simulink model "Model_6DOF"  (R2022a)
settings: Solver=FixedStepAuto  StartTime=0.0  StopTime=Tf  FixedStep=0.05  RelTol=1e-3
values from neighbouring files (symbols this model uses):
  Ba_0 = [0 0 0 0 0 0]    [run.m]
  Bv_0 = [-5.14444 0 0 0 0 0]    [run.m]
  Bx_0 = [0 0 -20 0 0 0]    [run.m]
  psi_ref = 0    [run.m]
  Seastate = 0    [run.m]
  Tf = 5000    [run.m]
  v_ref = Bv_0(1)    [run.m]
  z_ref = Bx_0(3)    [run.m]
undefined symbols (not defined in the file or in its folder): Bb, Cp, Cp_prime, dA_BP1, dA_BP2, dA_Hull, dA_PH, dA_Sail, dA_SProot, dA_X1a, dA_X1b, dA_X2a, dA_X2b, dA_X3a, dA_X3b, dA_X4a, dA_X4b, Ixx, Ixy, Ixz, Iyy, Iyz, Izz, Mb, n_BP1, n_BP2, n_Hull, n_PH, n_Sail, n_SProot, n_X2a, n_X2b, n_X3a, n_X4a, n_X4b, nt_BP1, nt_BP2, nt_Hull, nt_PH, nt_Sail, nt_SProot, nt_X1a, nt_X1b, nt_X2a, nt_X2b, nt_X3a, nt_X3b, nt_X4a, nt_X4b, tknots, vt1_BP1, vt1_BP2, vt1_Hull, vt1_PH, vt1_Sail, vt1_SProot, vt1_X1a, vt1_X1b, vt1_X2a, vt1_X2b ... (+39)
libraries: simulink x8
(part 2 of 5)

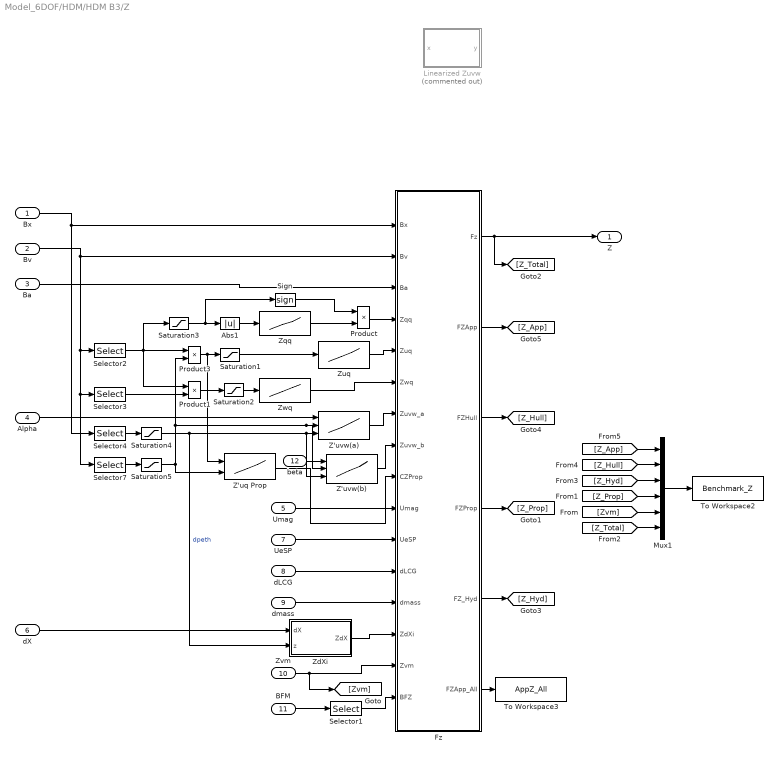
== system Model_6DOF/HDM/HDM B3/Z ==
  Bx : Inport
  Bv : Inport  Port=2
  Ba : Inport  Port=3
  Alpha : Inport  Port=4
  Umag : Inport  Port=5
  dX : Inport  Port=6
  UeSP : Inport  Port=7
  dLCG : Inport  Port=8
  dmass : Inport  Port=9
  Zvm : Inport  Port=10
  BFM : Inport  Port=11
  beta : Inport  Port=12
  Abs1 : Abs  SaturateOnIntegerOverflow=off
  Fz : MATLAB Function  TreatAsAtomicUnit=on
  Linearized Zuvw : MATLAB Function  Commented=on  TreatAsAtomicUnit=on
  Mux1 : Mux  Inputs=6
  Product : Product
  Product1 : Product
  Product3 : Product
  Saturation1 : Saturate  UpperLimit=0.04  LowerLimit=-0.04
  Saturation2 : Saturate  UpperLimit=0.0015  LowerLimit=-0.0015
  Saturation3 : Saturate  UpperLimit=0.02  LowerLimit=-0.02
  Saturation4 : Saturate  UpperLimit=-13.8724  LowerLimit=-35.0624
  Saturation5 : Saturate  UpperLimit=-1.5433E+00  LowerLimit=-5.14444
  Selector1 : Selector  InputPortWidth=6  IndexOptions=Index vector (dialog)  Indices=3  OutputSizes=1
  Selector2 : Selector  InputPortWidth=6  IndexOptions=Index vector (dialog)  Indices=5  OutputSizes=1
  Selector3 : Selector  InputPortWidth=6  IndexOptions=Index vector (dialog)  Indices=3  OutputSizes=1
  Selector4 : Selector  InputPortWidth=6  IndexOptions=Index vector (dialog)  Indices=3  OutputSizes=1
  Selector7 : Selector  InputPortWidth=6  IndexOptions=Index vector (dialog)  Indices=1  OutputSizes=1
  Sign : Signum
  To Workspace2 : ToWorkspace  VariableName=Benchmark_Z  SaveFormat=Timeseries  SampleTime=-1
  To Workspace3 : ToWorkspace  VariableName=AppZ_All  SaveFormat=Timeseries  SampleTime=-1
  Z'uq Prop : Lookup_n-D  BreakpointsForDimension1=|  BreakpointsForDimension2=[-7.71666 -5.14444 -3.086664 -1.543332]  Table=|  InternalRulePriority=Speed  RndMeth=Simplest
      BreakpointsForDimension1=|
      | [-2.0E-01
      | -1.5E-01
      | -1.0E-01
      | -5.0E-02
      | 0.0E+00
      | 5.0E-02
      | 1.0E-01
      | 1.5E-01
      | 2.0E-01
      | ]
      Table=|
      | reshape([1.3913E-04
      | 1.0452E-04
      | 6.9900E-05
      | 3.5283E-05
      | 6.6700E-07
      | -3.3949E-05
      | -6.8566E-05
      | -1.0318E-04
      | -1.3780E-04
      | 2.8914E-04
      | 2.1702E-04
      | 1.4490E-04
      | 7.2785E-05
      | 6.6700E-07
      | -7.1451E-05
      | -1.4357E-04
      | -2.1569E-04
      | -2.8780E-04
      | 1.1606E-04
      | 8.7208E-05
      | 5.8361E-05
      | 2.9514E-05
      | 6.6700E-07
      | -2.8180E-05
      | -5.7027E-05
      | -8.5874E-05
      | -1.1472E-04
      | 1.1606E-04
      | 8.7208E-05
      | 5.8361E-05
      | 2.9514E-05
      | 6.6700E-07
      | -2.8180E-05
      | -5.7027E-05
      | -8.5874E-05
      | -1.1472E-04],[9,4])
      settings: InputPortMap=u0,u1
  Z'uvw(a) : Lookup_n-D  NumberOfTableDimensions=3  BreakpointsForDimension1=|  BreakpointsForDimension2=|  BreakpointsForDimension3=|  Table=|  InternalRulePriority=Speed  RndMeth=Simplest
      BreakpointsForDimension1=|
      | [-12
      | -8
      | -4
      | 0
      | 4
      | 8
      | 12]
      BreakpointsForDimension2=|
      | [-5.1444E+00
      | -3.0866E+00
      | -1.5433E+00
      | ]
      Table=|
      | reshape([-3.82587E-03
      | -2.42543E-03
      | -1.05453E-03
      | 1.94202E-04
      | 1.48991E-03
      | 3.04047E-03
      | 4.14104E-03
      | -3.76348E-03
      | -2.38508E-03
      | -9.82619E-04
      | 1.94202E-04
      | 1.47560E-03
      | 3.02863E-03
      | 4.06663E-03
      | -3.75964E-03
      | -2.29001E-03
      | -8.34074E-04
      | 1.94202E-04
      | 1.38956E-03
      | 2.91153E-03
      | 4.15251E-03
      | -3.11218E-03
      | -1.80502E-03
      | -4.97855E-04
      | 8.09305E-04
      | 2.11647E-03
      | 3.42363E-03
      | 4.73079E-03
      | -2.62573E-03
      | -1.48072E-03
      | -3.35708E-04
      | 8.09305E-04
      | 1.95432E-03
      | 3.09933E-03
      | 4.24434E-03
      | -2.06413E-03
      | -1.10632E-03
      | -1.48507E-04
      | 8.09305E-04
      | 1.76712E-03
      | 2.72493E-03
      | 3.68274E-03
      | -3.09997E-03
      | -1.76300E-03
      | -4.26025E-04
      | 9.10947E-04
      | 2.24792E-03
      | 3.58489E-03
      | 4.92186E-03
      | -2.49055E-03
      | -1.35672E-03
      | -2.22886E-04
      | 9.10947E-04
      | 2.04478E-03
      | 3.17861E-03
      | 4.31245E-03
      | -2.64104E-03
      | -1.45704E-03
      | -2.73048E-04
      | 9.10947E-04
      | 2.09494E-03
      | 3.27894E-03
      | 4.46293E-03
      | -0.003059752
      | -0.001711935
      | -0.000364117
      | 0.0009837
      | 0.002331518
      | 0.003679335
      | 0.005027153
      | -0.002351082
      | -0.0012256
      | -0.000100118
      | 0.0009837
      | 0.002109182
      | 0.003234664
      | 0.004360146
      | -0.001725739
      | -0.000822593
      | 8.05539E-05
      | 0.0009837
      | 0.001886847
      | 0.002789993
      | 0.00369314],[7,3,4])
      BreakpointsForDimension3=|
      | [-35.0624 -18.3724 -15.3724 -13.8724
      | ]
      settings: InputPortMap=u0,u1,u2
  Z'uvw(b) : Lookup_n-D  NumberOfTableDimensions=3  BreakpointsForDimension1=|  BreakpointsForDimension2=|  BreakpointsForDimension3=|  Table=|  InternalRulePriority=Speed  RndMeth=Simplest
      BreakpointsForDimension1=|
      | [0
      | 4
      | 8
      | 12]
      BreakpointsForDimension2=|
      | [-5.1444E+00
      | -3.0866E+00
      | -1.5433E+00
      | ]
      Table=|
      | reshape([0.0000000E+00
      | -5.9986916E-04
      | -2.7503348E-03
      | -5.0777589E-03
      | 0.0000000E+00
      | -6.0654884E-04
      | -2.4512564E-03
      | -5.2464901E-03
      | 0.0000000E+00
      | -7.6137528E-04
      | -2.4084463E-03
      | -5.2118678E-03
      | 0.0000000E+00
      | -8.2427914E-04
      | -2.5250249E-03
      | -5.3103563E-03
      | 0.0000000E+00
      | -8.1036019E-04
      | -2.5315266E-03
      | -5.5141459E-03
      | 0.0000000E+00
      | -7.9799041E-04
      | -2.5595242E-03
      | -5.2319004E-03
      | 0.0000000E+00
      | -8.6989011E-04
      | -2.5865820E-03
      | -5.6151595E-03
      | 0.0000000E+00
      | -8.4361582E-04
      | -2.6124115E-03
      | -5.7143353E-03
      | 0.0000000E+00
      | -8.2567611E-04
      | -2.6088331E-03
      | -5.6150660E-03
      | 0.0000000E+00
      | -9.1003224E-04
      | -2.7683191E-03
      | -6.0189061E-03
      | 0.0000000E+00
      | -8.4211433E-04
      | -2.5899187E-03
      | -5.7497784E-03
      | 0.0000000E+00
      | -8.2014014E-04
      | -2.4092466E-03
      | -5.6643347E-03],[4,3,4])
      BreakpointsForDimension3=|
      | [-35.0624 -18.3724 -15.3724 -13.8724
      | ]
      settings: InputPortMap=u0,u1,u2
  ZdXi : Subsystem
  Zqq : Lookup_n-D  NumberOfTableDimensions=1  BreakpointsForDimension1=|  Table=|  InternalRulePriority=Speed  RndMeth=Simplest
      BreakpointsForDimension1=|
      | [0.000127901
      | 0.000383704
      | 0.000639507
      | 0.001279013
      | 0.002558026
      | ]
      Table=|
      | [-1.5611E-03
      | -1.0379E-04
      | 3.9238E-05
      | 1.1475E-04
      | 1.3579E-04
      | ]
  Zuq : Lookup_n-D  NumberOfTableDimensions=1  BreakpointsForDimension1=|  Table=|  InternalRulePriority=Speed  RndMeth=Simplest
      BreakpointsForDimension1=|
      | [-0.04
      | -0.03
      | -0.02
      | -0.01
      | -0.005
      | -0.002
      | 0.002
      | 0.005
      | 0.01
      | 0.02
      | 0.03
      | 0.04
      | ]
      Table=|
      | [-9.8908E-03
      | -9.0784E-03
      | -8.9566E-03
      | -1.0733E-02
      | -1.4141E-02
      | -2.4189E-02
      | -6.5605E-03
      | -7.1594E-03
      | -7.6366E-03
      | -7.9008E-03
      | -6.1794E-03
      | -6.1029E-03
      | ]
  Zwq : Lookup_n-D  NumberOfTableDimensions=1  BreakpointsForDimension1=|  Table=|  InternalRulePriority=Speed  RndMeth=Simplest
      BreakpointsForDimension1=|
      | [-0.0015
      | -0.0012
      | -0.0009
      | -0.0006
      | -0.0003
      | -0.0001
      | 0.0001
      | 0.0003
      | 0.0006
      | 0.0009
      | 0.0012
      | 0.0015]
      Table=|
      | [-2.9784E-01
      | -2.6725E-01
      | -2.3292E-01
      | -2.0077E-01
      | -1.1489E-01
      | -7.6673E-03
      | -7.5516E-03
      | -1.1617E-01
      | -2.0077E-01
      | -2.9128E-01
      | -3.5974E-01
      | -4.7839E-01]
  Z : Outport
  wires:
  Selector4/1 -> Saturation4/1
  Zvm/1 -> Fz/15(Zvm), [Zvm]
  Ba/1 -> Fz/3(Ba)
  Zuq/1 -> Fz/5(Zuq)
  Fz/1(Fz) -> Z/1, [Z_Total]
  Saturation3/1 -> Abs1/1, Sign/1
  Saturation2/1 -> Zwq/1
  Saturation1/1 -> Zuq/1
  dX/1 -> ZdXi/1(dX)
  dmass/1 -> Fz/13(dmass)
  dLCG/1 -> Fz/12(dLCG)
  Product1/1 -> Saturation2/1
  Selector3/1 -> Product1/2
  UeSP/1 -> Fz/11(UeSP)
  Product3/1 -> Saturation1/1, Z'uq Prop/1
  Bx/1 -> Fz/1(Bx), Selector4/1
  Umag/1 -> Fz/10(Umag)
  Bv/1 -> Fz/2(Bv), Selector2/1, Selector3/1, Selector7/1
  Alpha/1 -> Z'uvw(a)/1
  Selector2/1 -> Product3/1, Product1/1, Saturation3/1
  Zwq/1 -> Fz/6(Zwq)
  Z'uq Prop/1 -> Fz/9(CZProp)
  Zqq/1 -> Product/2
  Z'uvw(a)/1 -> Fz/7(Zuvw_a)
  BFM/1 -> Selector1/1
  Selector1/1 -> Fz/16(BFZ)
  ZdXi/1(ZdX) -> Fz/14(ZdXi)
  [Z_Hull] -> Mux1/2
  [Z_App] -> Mux1/1
  Mux1/1 -> To Workspace2/1
  [Z_Prop] -> Mux1/4
  [Z_Total] -> Mux1/6
  [Z_Hyd] -> Mux1/3
  [Zvm] -> Mux1/5
  Fz/2(FZApp) -> [Z_App]
  Fz/3(FZHull) -> [Z_Hull]
  Fz/4(FZProp) -> [Z_Prop]
  Fz/5(FZ_Hyd) -> [Z_Hyd]
  Saturation4/1 -> Z'uvw(b)/3, Z'uvw(a)/3, ZdXi/2(z)  "dpeth"
  Saturation5/1 -> Product3/2, Z'uvw(a)/2, Z'uvw(b)/2, Z'uq Prop/2
  Selector7/1 -> Saturation5/1
  Fz/6(FZApp_All) -> To Workspace3/1
  Abs1/1 -> Zqq/1
  Sign/1 -> Product/1
  Product/1 -> Fz/4(Zqq)
  Z'uvw(b)/1 -> Fz/8(Zuvw_b)
  beta/1 -> Z'uvw(b)/1

== system Model_6DOF/HDM/Integration and Coord. Transfrom/Coordinate Transform ==
  Bv : Inport
  Integrator : Integrator  InitialCondition=Bx_0
  MATLAB Function2 : MATLAB Function  TreatAsAtomicUnit=on
  X_earth : Outport  VectorParamsAs1DForOutWhenUnconnected=off
  wires:
  Bv/1 -> MATLAB Function2/2(Bv)
  MATLAB Function2/1(out) -> Integrator/1
  Integrator/1 -> X_earth/1, MATLAB Function2/1(Bx)

== system Model_6DOF/HDM/Integration and Coord. Transfrom/Rigid Body Motion ==
  F_hyd : Inport
  Bx : Inport  Port=2
  Demux : Demux  Outputs=6
  Demux1 : Demux  Outputs=6
  Demux2 : Demux  Outputs=5
  Gain2 : Gain
  Integrator : Integrator  InitialCondition=Bv_0
  MATLAB Function2 : MATLAB Function  TreatAsAtomicUnit=on
  Memory1 : Memory  InitialCondition=Ba_0
  Mux1 : Mux  Inputs=6
  Mux2 : Mux  Inputs=5
  Bv : Outport  VectorParamsAs1DForOutWhenUnconnected=off
  Ba : Outport  Port=2  VectorParamsAs1DForOutWhenUnconnected=off
  wires:
  Bx/1 -> MATLAB Function2/7(bx)
  MATLAB Function2/1(out) -> Integrator/1, Memory1/1
  Integrator/1 -> MATLAB Function2/8(bv), Demux1/1
  Memory1/1 -> Ba/1
  Demux/1 -> MATLAB Function2/1(X)
  Demux/2 -> MATLAB Function2/2(Y)
  Demux/3 -> MATLAB Function2/3(Z)
  Demux/4 -> MATLAB Function2/4(K)
  Demux/5 -> MATLAB Function2/5(M)
  Demux/6 -> MATLAB Function2/6(N)
  F_hyd/1 -> Demux/1
  Demux2/3 -> Mux1/4
  Demux1/3 -> Mux2/2
  Mux2/1 -> Gain2/1
  Demux2/5 -> Mux1/6
  Demux2/2 -> Mux1/3
  Demux2/4 -> Mux1/5
  Demux1/1 -> Mux1/1
  Demux2/1 -> Mux1/2
  Demux1/5 -> Mux2/4
  Demux1/6 -> Mux2/5
  Demux1/4 -> Mux2/3
  Demux1/2 -> Mux2/1
  Gain2/1 -> Demux2/1
  Mux1/1 -> Bv/1

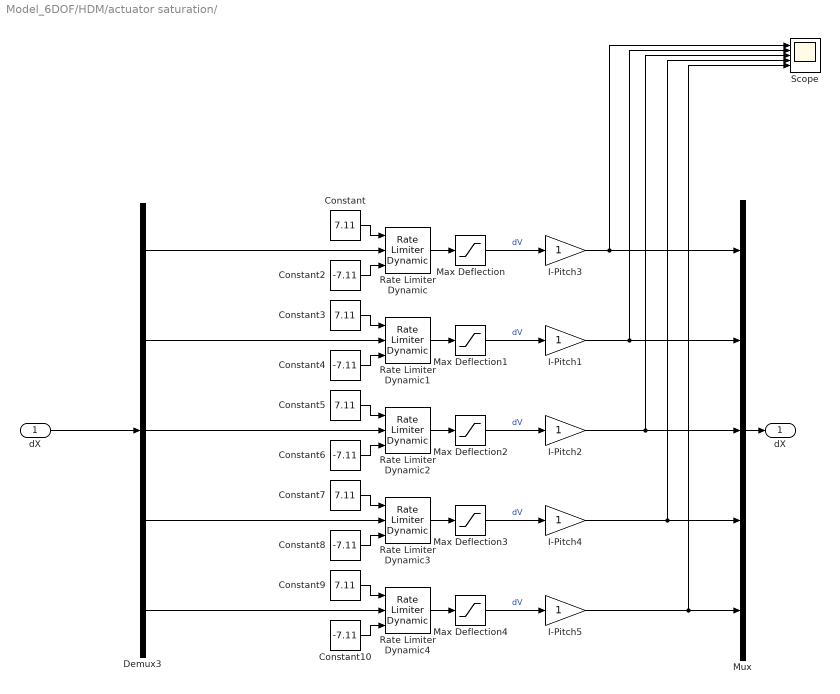
== system Model_6DOF/HDM/actuator saturation/  ==
  "dX " : Inport
  Constant{,3,5,7,9} (5 alike) : Constant  Value=7.11
  Constant{2,4,6,8,10} (5 alike) : Constant  Value=-7.11
  Demux3 : Demux  Outputs=5
  I-Pitch{1..5} (5 alike) : Gain
  Max Deflection{,1..4} (5 alike) : Saturate  UpperLimit=30  LowerLimit=-30
  Mux : Mux  Inputs=5
  Rate Limiter Dynamic{,1..4} (5 alike) : simulink/Discontinuities/Rate Limiter Dynamic
  Scope : Scope  NumInputPorts=5
  dX : Outport
  wires:
  I-Pitch2/1 -> Scope/3, Mux/3
  Constant2/1 -> Rate Limiter Dynamic/3
  Constant9/1 -> Rate Limiter Dynamic4/1
  Demux3/1 -> Rate Limiter Dynamic/2
  Max Deflection/1 -> I-Pitch3/1  "dV"
  Demux3/3 -> Rate Limiter Dynamic2/2
  Demux3/5 -> Rate Limiter Dynamic4/2
  Constant3/1 -> Rate Limiter Dynamic1/1
  Demux3/4 -> Rate Limiter Dynamic3/2
  Demux3/2 -> Rate Limiter Dynamic1/2
  Constant10/1 -> Rate Limiter Dynamic4/3
  Rate Limiter Dynamic/1 -> Max Deflection/1
  I-Pitch5/1 -> Scope/5, Mux/5
  Rate Limiter Dynamic4/1 -> Max Deflection4/1
  Max Deflection2/1 -> I-Pitch2/1  "dV"
  I-Pitch1/1 -> Scope/2, Mux/2
  Constant4/1 -> Rate Limiter Dynamic1/3
  I-Pitch3/1 -> Scope/1, Mux/1
  I-Pitch4/1 -> Scope/4, Mux/4
  Constant6/1 -> Rate Limiter Dynamic2/3
  Rate Limiter Dynamic1/1 -> Max Deflection1/1
  Constant/1 -> Rate Limiter Dynamic/1
  Rate Limiter Dynamic2/1 -> Max Deflection2/1
  Max Deflection1/1 -> I-Pitch1/1  "dV"
  Constant5/1 -> Rate Limiter Dynamic2/1
  Max Deflection3/1 -> I-Pitch4/1  "dV"
  "dX "/1 -> Demux3/1
  Constant8/1 -> Rate Limiter Dynamic3/3
  Max Deflection4/1 -> I-Pitch5/1  "dV"
  Constant7/1 -> Rate Limiter Dynamic3/1
  Mux/1 -> dX/1
  Rate Limiter Dynamic3/1 -> Max Deflection3/1

== system Model_6DOF/HDM/actuator saturation/    ==
  "n " : Inport
  Rate Limiter Dynamic : simulink/Discontinuities/Rate Limiter Dynamic
  Rate Max : Constant  Value=14.65
  Rate Min : Constant  Value=-14.65
  Saturation6 : Saturate  UpperLimit=10  LowerLimit=0.01
  n : Outport
  wires:
  "n "/1 -> Rate Limiter Dynamic/2
  Rate Min/1 -> Rate Limiter Dynamic/3
  Rate Limiter Dynamic/1 -> Saturation6/1
  Rate Max/1 -> Rate Limiter Dynamic/1
  Saturation6/1 -> n/1

== system Model_6DOF/HDM/actuator saturation/Subsystem1 ==
  dLCG : Inport
  " LCG Change Saturation" : Saturate
  Lower Rate limit : Constant  Value=-5.83e-4
  Rate Limiter Dynamic : simulink/Discontinuities/Rate Limiter Dynamic
  Upper Rate limit : Constant  Value=5.83e-4
  dLCG (m) : Outport
  wires:
  " LCG Change Saturation"/1 -> dLCG (m)/1  "dLCG (m)"
  Rate Limiter Dynamic/1 -> " LCG Change Saturation"/1  "dLCG (m)"
  Lower Rate limit/1 -> Rate Limiter Dynamic/3
  Upper Rate limit/1 -> Rate Limiter Dynamic/1
  dLCG/1 -> Rate Limiter Dynamic/2

== system Model_6DOF/HDM/actuator saturation/Subsystem2 ==
  dmass : Inport
  Constant2 : Constant  Value=100
  Constant3 : Constant  Value=-100
  Max Mass Change : Saturate  UpperLimit=20000  LowerLimit=-20000
  Rate Limiter Dynamic1 : simulink/Discontinuities/Rate Limiter Dynamic
  dmass (kg) : Outport
  wires:
  Constant3/1 -> Rate Limiter Dynamic1/3
  Rate Limiter Dynamic1/1 -> Max Mass Change/1  "dmass (kg)"
  Constant2/1 -> Rate Limiter Dynamic1/1
  dmass/1 -> Rate Limiter Dynamic1/2
  Max Mass Change/1 -> dmass (kg)/1  "dmass (kg)"

== system Model_6DOF/HDM/HDM B3/K/KdXi ==
  dX : Inport
  UeX : Inport  Port=2
  z : Inport  Port=3
  KdX1 : Lookup_n-D  NumberOfTableDimensions=3  BreakpointsForDimension1=[-10 0 10]  BreakpointsForDimension2=|  BreakpointsForDimension3=[-5.14444 -3.08666664 -1.54332]  Table=|  InternalRulePriority=Speed  RndMeth=Simplest
      BreakpointsForDimension2=|
      | [-36.4062987
      | -18.4062987
      | -15.4062987
      | -13.9062987]
      Table=|
      | reshape([-3.9047E-05
      | 4.5684E-07
      | 3.9769E-05
      | -3.8309E-05
      | 1.2643E-06
      | 4.0809E-05
      | -3.0256E-05
      | 1.2643E-06
      | 4.8387E-05
      | -3.7558E-05
      | 2.1545E-06
      | 4.2083E-05
      | -3.9057E-05
      | 3.6064E-07
      | 3.9562E-05
      | -3.8473E-05
      | 1.0476E-06
      | 4.0437E-05
      | -3.0256E-05
      | 1.4418E-06
      | 4.8387E-05
      | -3.7906E-05
      | 1.7415E-06
      | 4.1434E-05
      | -3.8945E-05
      | 2.8249E-07
      | 3.9429E-05
      | -3.8396E-05
      | 9.1134E-07
      | 4.0237E-05
      | -3.8190E-05
      | 9.1134E-07
      | 4.0733E-05
      | -3.7932E-05
      | 1.5343E-06
      | 4.1020E-05
      | ],[3,4,3])
      settings: InputPortMap=u0,u1,u2
  KdX2 : Lookup_n-D  NumberOfTableDimensions=3  BreakpointsForDimension1=[-10 0 10]  BreakpointsForDimension2=|  BreakpointsForDimension3=[-5.14444 -3.08666664 -1.54332]  Table=|  InternalRulePriority=Speed  RndMeth=Simplest
      BreakpointsForDimension2=|
      | [-36.4062987
      | -18.4062987
      | -15.4062987
      | -13.9062987]
      Table=|
      | reshape([-3.5775E-05
      | -2.4080E-07
      | 3.3150E-05
      | -3.4263E-05
      | 1.2268E-06
      | 3.5342E-05
      | -2.3577E-05
      | 1.2268E-06
      | 4.6338E-05
      | -3.2368E-05
      | 3.5682E-06
      | 3.9469E-05
      | -3.5785E-05
      | -3.3131E-07
      | 3.3067E-05
      | -3.4544E-05
      | 8.9010E-07
      | 3.4889E-05
      | -2.3577E-05
      | 1.7076E-06
      | 4.6338E-05
      | -3.3141E-05
      | 2.4187E-06
      | 3.7389E-05
      | -3.5809E-05
      | -5.7189E-07
      | 3.3046E-05
      | -3.4706E-05
      | 4.2723E-07
      | 3.4588E-05
      | -3.4017E-05
      | 4.2723E-07
      | 3.5657E-05
      | -3.3562E-05
      | 1.6134E-06
      | 3.6605E-05
      | ],[3,4,3])
      settings: InputPortMap=u0,u1,u2
  KdX3 : Lookup_n-D  NumberOfTableDimensions=3  BreakpointsForDimension1=[-10 0 10]  BreakpointsForDimension2=|  BreakpointsForDimension3=[-5.14444 -3.08666664 -1.54332]  Table=|  InternalRulePriority=Speed  RndMeth=Simplest
      BreakpointsForDimension2=|
      | [-36.4062987
      | -18.4062987
      | -15.4062987
      | -13.9062987]
      Table=|
      | reshape([-4.3139E-05
      | 1.7292E-07
      | 4.5001E-05
      | -4.4081E-05
      | -1.2796E-06
      | 4.2448E-05
      | -4.9749E-05
      | -1.2796E-06
      | 2.6691E-05
      | -4.5613E-05
      | -3.5861E-06
      | 3.8362E-05
      | -4.2707E-05
      | 2.7384E-07
      | 4.4575E-05
      | -4.3360E-05
      | -9.3523E-07
      | 4.2465E-05
      | -4.9749E-05
      | -1.7362E-06
      | 2.6691E-05
      | -4.4279E-05
      | -2.4363E-06
      | 3.9821E-05
      | -4.1687E-05
      | 5.3371E-07
      | 4.3082E-05
      | -4.2289E-05
      | -4.5361E-07
      | 4.1207E-05
      | -4.2616E-05
      | -4.5361E-07
      | 4.0204E-05
      | -4.2521E-05
      | -1.6159E-06
      | 3.9463E-05
      | ],[3,4,3])
      settings: InputPortMap=u0,u1,u2
  KdX4 : Lookup_n-D  NumberOfTableDimensions=3  BreakpointsForDimension1=[-10 0 10]  BreakpointsForDimension2=|  BreakpointsForDimension3=[-5.14444 -3.08666664 -1.54332]  Table=|  InternalRulePriority=Speed  RndMeth=Simplest
      BreakpointsForDimension2=|
      | [-36.4062987
      | -18.4062987
      | -15.4062987
      | -13.9062987]
      Table=|
      | reshape([-4.0969E-05
      | -4.5313E-07
      | 4.0019E-05
      | -4.1787E-05
      | -1.2714E-06
      | 3.9006E-05
      | -4.8908E-05
      | -1.2714E-06
      | 3.0663E-05
      | -4.2681E-05
      | -2.1920E-06
      | 3.7920E-05
      | -4.0777E-05
      | -3.6185E-07
      | 4.0047E-05
      | -4.1470E-05
      | -1.0577E-06
      | 3.9147E-05
      | -4.8908E-05
      | -1.4679E-06
      | 3.0663E-05
      | -4.2187E-05
      | -1.7779E-06
      | 3.8312E-05
      | -4.0496E-05
      | -2.8854E-07
      | 4.0049E-05
      | -4.1082E-05
      | -9.2714E-07
      | 3.9223E-05
      | -4.1472E-05
      | -9.2714E-07
      | 3.8784E-05
      | -4.1733E-05
      | -1.5768E-06
      | 3.8383E-05
      | ],[3,4,3])
      settings: InputPortMap=u0,u1,u2
  Mux : Mux
  Selector1 : Selector  InputPortWidth=5  IndexOptions=Index vector (dialog)  Indices=2  OutputSizes=1
  Selector2 : Selector  InputPortWidth=5  IndexOptions=Index vector (dialog)  Indices=3  OutputSizes=1
  Selector3 : Selector  InputPortWidth=5  IndexOptions=Index vector (dialog)  Indices=4  OutputSizes=1
  Selector4 : Selector  InputPortWidth=5  IndexOptions=Index vector (dialog)  Indices=1  OutputSizes=1
  Selector5 : Selector  InputPortWidth=5  IndexOptions=Index vector (dialog)  Indices=2  OutputSizes=1
  Selector6 : Selector  InputPortWidth=5  IndexOptions=Index vector (dialog)  Indices=3  OutputSizes=1
  Selector7 : Selector  InputPortWidth=5  IndexOptions=Index vector (dialog)  Indices=1  OutputSizes=1
  Selector8 : Selector  InputPortWidth=5  IndexOptions=Index vector (dialog)  Indices=4  OutputSizes=1
  KdXi : Outport
  wires:
  dX/1 -> Selector1/1, Selector3/1, Selector2/1, Selector7/1
  Selector7/1 -> KdX1/1
  Mux/1 -> KdXi/1
  z/1 -> KdX4/2, KdX3/2, KdX2/2, KdX1/2
  KdX1/1 -> Mux/1
  KdX2/1 -> Mux/2
  KdX3/1 -> Mux/3
  KdX4/1 -> Mux/4
  Selector1/1 -> KdX2/1
  Selector2/1 -> KdX3/1
  Selector3/1 -> KdX4/1
  UeX/1 -> Selector6/1, Selector8/1, Selector5/1, Selector4/1
  Selector4/1 -> KdX1/3
  Selector8/1 -> KdX4/3
  Selector6/1 -> KdX3/3
  Selector5/1 -> KdX2/3

== system Model_6DOF/HDM/HDM B3/M/Mdxi ==
  dX : Inport
  z : Inport  Port=2
  Demux6 : Demux  Outputs=5
  Gain{,1..4} (5 alike) : Gain
  Mux : Mux  Inputs=5
  ZudX1 q+1 : Lookup_n-D  BreakpointsForDimension1=[-30 -20 -10 0 10 20 30]  BreakpointsForDimension2=[-35.0624 -15.3724 -13.8724]  BreakpointsForDimension3=[-5.14444 -3.08666664 -1.54332]  Table=|  InternalRulePriority=Speed  RndMeth=Simplest
      | reshape([0.000594819
      | 0.000394915
      | 0.000195011
      | -4.89222E-06
      | -0.000204796
      | -0.0004047
      | -0.000604603
      | 0.000596203
      | 0.000392018
      | 0.000187833
      | -1.6352E-05
      | -0.000220537
      | -0.000424722
      | -0.000628907
      | 0.000582351
      | 0.000381446
      | 0.000180542
      | -2.03625E-05
      | -0.000221267
      | -0.000422171
      | -0.000623076
      | ],[7,3])
      settings: InputPortMap=u0,u1
  ZudX1 q+2 : Lookup_n-D  BreakpointsForDimension1=[-30 -20 -10 0 10 20 30]  BreakpointsForDimension2=[-35.0624 -15.3724 -13.8724]  BreakpointsForDimension3=[-5.14444 -3.08666664 -1.54332]  Table=|  InternalRulePriority=Speed  RndMeth=Simplest
      | reshape([0.000583784
      | 0.000394316
      | 0.000204847
      | 1.53782E-05
      | -0.000174091
      | -0.000363559
      | -0.000553028
      | 0.00056228
      | 0.000374724
      | 0.000187169
      | -3.86644E-07
      | -0.000187942
      | -0.000375498
      | -0.000563053
      | 0.000546298
      | 0.000362052
      | 0.000177806
      | -6.43933E-06
      | -0.000190685
      | -0.000374931
      | -0.000559176],[7,3])
      settings: InputPortMap=u0,u1
  ZudX1 q+3 : Lookup_n-D  BreakpointsForDimension1=[-30 -20 -10 0 10 20 30]  BreakpointsForDimension2=[-35.0624 -15.3724 -13.8724]  BreakpointsForDimension3=[-5.14444 -3.08666664 -1.54332]  Table=|  InternalRulePriority=Speed  RndMeth=Simplest
      | reshape([-0.000586989
      | -0.000395541
      | -0.000204094
      | -1.26467E-05
      | 0.000178801
      | 0.000370248
      | 0.000561695
      | -0.000568868
      | -0.000379268
      | -0.000189669
      | -6.86388E-08
      | 0.000189531
      | 0.000379131
      | 0.000568731
      | -0.000565299
      | -0.000378949
      | -0.000192598
      | -6.24776E-06
      | 0.000180103
      | 0.000366453
      | 0.000552804],[7,3])
      settings: InputPortMap=u0,u1
  ZudX1 q+4 : Lookup_n-D  BreakpointsForDimension1=[-30 -20 -10 0 10 20 30]  BreakpointsForDimension2=[-35.0624 -15.3724 -13.8724]  BreakpointsForDimension3=[-5.14444 -3.08666664 -1.54332]  Table=|  InternalRulePriority=Speed  RndMeth=Simplest
      | reshape([-0.000638396
      | -0.000426715
      | -0.000215035
      | -3.35454E-06
      | 0.000208326
      | 0.000420006
      | 0.000631687
      | -0.000598951
      | -0.000393944
      | -0.000188937
      | 1.60698E-05
      | 0.000221077
      | 0.000426084
      | 0.000631091
      | -0.000622514
      | -0.000421726
      | -0.000220939
      | -2.01522E-05
      | 0.000180635
      | 0.000381422
      | 0.000582209],[7,3])
      settings: InputPortMap=u0,u1
  ZudX1 q+5 : Lookup_n-D  BreakpointsForDimension1=[-30 -20 -10 0 10 20 30]  BreakpointsForDimension2=[-35.0624 -15.3724 -13.8724]  BreakpointsForDimension3=[-35.0624 -15.3724 -13.8724]  Table=|  InternalRulePriority=Speed  RndMeth=Simplest
      | reshape([-0.000461714
      | -0.000296336
      | -0.000130959
      | 3.44194E-05
      | 0.000199797
      | 0.000365175
      | 0.000530553
      | -0.000503641
      | -0.000327652
      | -0.000151663
      | 2.43257E-05
      | 0.000200315
      | 0.000376303
      | 0.000552292
      | -0.000536558
      | -0.000356664
      | -0.00017677
      | 3.1235E-06
      | 0.000183017
      | 0.000362911
      | 0.000542805],[7,3])
      settings: InputPortMap=u0,u1
  MdX : Outport
  wires:
  Demux6/5 -> ZudX1 q+5/1
  Demux6/4 -> ZudX1 q+4/1
  Demux6/3 -> ZudX1 q+3/1
  Demux6/2 -> ZudX1 q+2/1
  ZudX1 q+4/1 -> Gain1/1
  ZudX1 q+3/1 -> Gain2/1
  ZudX1 q+2/1 -> Gain3/1
  ZudX1 q+1/1 -> Gain/1
  ZudX1 q+5/1 -> Gain4/1
  z/1 -> ZudX1 q+5/2, ZudX1 q+4/2, ZudX1 q+3/2, ZudX1 q+2/2, ZudX1 q+1/2
  Mux/1 -> MdX/1
  Demux6/1 -> ZudX1 q+1/1
  dX/1 -> Demux6/1
  Gain/1 -> Mux/1
  Gain3/1 -> Mux/2
  Gain2/1 -> Mux/3
  Gain1/1 -> Mux/4
  Gain4/1 -> Mux/5

== system Model_6DOF/HDM/HDM B3/N/NdXi ==
  dX : Inport
  z : Inport  Port=2
  Mux : Mux
  NdX1 : Lookup_n-D  BreakpointsForDimension1=[-10 0 10]  BreakpointsForDimension2=|  BreakpointsForDimension3=[-5.14444 -3.08666664 -1.54332]  Table=|  InternalRulePriority=Speed  RndMeth=Simplest
      BreakpointsForDimension2=|
      | [-36.4062987
      | -18.4062987
      | -15.4062987
      | -13.9062987]
      Table=|
      | reshape([-8.13475E-05
      | -3.25752E-06
      | 6.9363E-05
      | -8.00129E-05
      | -1.7093E-06
      | 7.14001E-05
      | -6.46417E-05
      | -1.7093E-06
      | 8.57128E-05
      | -7.85432E-05
      | -1.19372E-08
      | 7.37459E-05],[3,4])
      settings: InputPortMap=u0,u1
  NdX2 : Lookup_n-D  BreakpointsForDimension1=[-10 0 10]  BreakpointsForDimension2=|  BreakpointsForDimension3=[-5.14444 -3.08666664 -1.54332]  Table=|  InternalRulePriority=Speed  RndMeth=Simplest
      BreakpointsForDimension2=|
      | [-36.4062987
      | -18.4062987
      | -15.4062987
      | -13.9062987]
      Table=|
      | reshape([6.2278E-05
      | -3.5277E-06
      | -7.1028E-05
      | 5.9473E-05
      | -6.2352E-06
      | -7.5067E-05
      | 3.9525E-05
      | -6.2352E-06
      | -9.4282E-05
      | 5.5892E-05
      | -1.0640E-05
      | -8.2654E-05],[3,4])
      settings: InputPortMap=u0,u1
  NdX3 : Lookup_n-D  BreakpointsForDimension1=[-10 0 10]  BreakpointsForDimension2=|  BreakpointsForDimension3=[-5.14444 -3.08666664 -1.54332]  Table=|  InternalRulePriority=Speed  RndMeth=Simplest
      BreakpointsForDimension2=|
      | [-36.4062987
      | -18.4062987
      | -15.4062987
      | -13.9062987]
      Table=|
      | reshape([8.96891E-05
      | 3.65995E-06
      | -8.07998E-05
      | 9.13096E-05
      | 6.34009E-06
      | -7.59117E-05
      | 0.000100356
      | 6.34009E-06
      | -4.56822E-05
      | 9.40576E-05
      | 1.06795E-05
      | -6.79415E-05],[3,4])
      settings: InputPortMap=u0,u1
  NdX4 : Lookup_n-D  BreakpointsForDimension1=[-10 0 10]  BreakpointsForDimension2=|  BreakpointsForDimension3=[-5.14444 -3.08666664 -1.54332]  Table=|  InternalRulePriority=Speed  RndMeth=Simplest
      BreakpointsForDimension2=|
      | [-36.4062987
      | -18.4062987
      | -15.4062987
      | -13.9062987]
      Table=|
      | reshape([-7.16232E-05
      | 3.25314E-06
      | 8.32589E-05
      | -7.3213E-05
      | 1.68586E-06
      | 8.13825E-05
      | -8.66615E-05
      | 1.68586E-06
      | 6.54218E-05
      | -7.48528E-05
      | -6.7812E-08
      | 7.92559E-05],[3,4])
      settings: InputPortMap=u0,u1
  Selector1 : Selector  InputPortWidth=5  IndexOptions=Index vector (dialog)  Indices=2  OutputSizes=1
  Selector2 : Selector  InputPortWidth=5  IndexOptions=Index vector (dialog)  Indices=3  OutputSizes=1
  Selector3 : Selector  InputPortWidth=5  IndexOptions=Index vector (dialog)  Indices=4  OutputSizes=1
  Selector7 : Selector  InputPortWidth=5  IndexOptions=Index vector (dialog)  Indices=1  OutputSizes=1
  NdXi : Outport
  wires:
  dX/1 -> Selector3/1, Selector2/1, Selector1/1, Selector7/1
  Selector7/1 -> NdX1/1
  Mux/1 -> NdXi/1
  z/1 -> NdX4/2, NdX3/2, NdX2/2, NdX1/2
  NdX1/1 -> Mux/1
  NdX2/1 -> Mux/2
  NdX3/1 -> Mux/3
  NdX4/1 -> Mux/4
  Selector1/1 -> NdX2/1
  Selector2/1 -> NdX3/1
  Selector3/1 -> NdX4/1

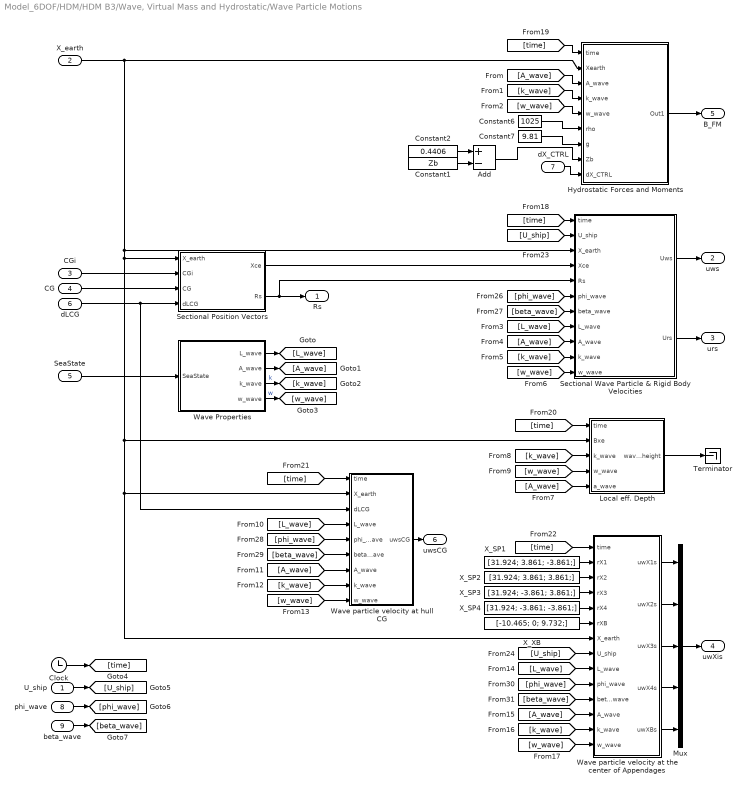
== system Model_6DOF/HDM/HDM B3/Wave, Virtual Mass and Hydrostatic/Wave Particle Motions ==
  U_ship : Inport
  X_earth : Inport  Port=2
  CGi : Inport  Port=3
  CG : Inport  Port=4
  SeaState : Inport  Port=5
  dLCG : Inport  Port=6
  dX_CTRL : Inport  Port=7
  phi_wave : Inport  Port=8
  beta_wave : Inport  Port=9
  Add : Sum  Inputs=+-
  Clock : Clock
  Constant1 : Constant  Value=Zb
  Constant2 : Constant  Value=0.4406
  Constant6 : Constant  Value=1025
  Constant7 : Constant  Value=9.81
  Hydrostatic Forces and Moments : Subsystem
  Local eff. Depth : MATLAB Function  TreatAsAtomicUnit=on
  Mux : Mux  Inputs=5
  Sectional Position Vectors : MATLAB Function  TreatAsAtomicUnit=on
  Sectional Wave Particle & Rigid Body Velocities : MATLAB Function  TreatAsAtomicUnit=on
  Terminator : Terminator
  Wave Properties : MATLAB Function  TreatAsAtomicUnit=on
  Wave particle velocity at hull CG : MATLAB Function  TreatAsAtomicUnit=on
  Wave particle velocity at the center of Appendages : MATLAB Function  TreatAsAtomicUnit=on
  X_SP1 : Constant  Value=[31.924; 3.861; -3.861;]
  X_SP2 : Constant  Value=[31.924; 3.861; 3.861;]
  X_SP3 : Constant  Value=[31.924; -3.861; 3.861;]
  X_SP4 : Constant  Value=[31.924; -3.861; -3.861;]
  X_XB : Constant  Value=[-10.465; 0; 9.732;]
  Rs : Outport
  uws : Outport  Port=2
  urs : Outport  Port=3
  uwXis : Outport  Port=4
  B_FM : Outport  Port=5
  uwsCG : Outport  Port=6
  wires:
  Sectional Position Vectors/2(Rs) -> Rs/1, Sectional Wave Particle & Rigid Body Velocities/5(Rs)
  SeaState/1 -> Wave Properties/1(SeaState)
  Sectional Position Vectors/1(Xce) -> Sectional Wave Particle & Rigid Body Velocities/4(Xce)
  X_earth/1 -> Wave particle velocity at hull CG/2(X_earth), Wave particle velocity at the center of Appendages/7(X_earth), Local eff. Depth/2(Bxe), Sectional Position Vectors/1(X_earth), Sectional Wave Particle & Rigid Body Velocities/3(X_earth), Hydrostatic Forces and Moments/2(Xearth)
  CGi/1 -> Sectional Position Vectors/2(CGi)
  CG/1 -> Sectional Position Vectors/3(CG)
  Sectional Wave Particle & Rigid Body Velocities/2(Urs) -> urs/1
  Sectional Wave Particle & Rigid Body Velocities/1(Uws) -> uws/1
  dLCG/1 -> Wave particle velocity at hull CG/3(dLCG), Sectional Position Vectors/4(dLCG)
  Local eff. Depth/1(wave_height) -> Terminator/1
  X_XB/1 -> Wave particle velocity at the center of Appendages/6(rXB)
  X_SP4/1 -> Wave particle velocity at the center of Appendages/5(rX4)
  X_SP3/1 -> Wave particle velocity at the center of Appendages/4(rX3)
  X_SP2/1 -> Wave particle velocity at the center of Appendages/3(rX2)
  X_SP1/1 -> Wave particle velocity at the center of Appendages/2(rX1)
  Wave particle velocity at the center of Appendages/1(uwX1s) -> Mux/1
  Wave particle velocity at the center of Appendages/2(uwX2s) -> Mux/2
  Wave particle velocity at the center of Appendages/3(uwX3s) -> Mux/3
  Wave particle velocity at the center of Appendages/4(uwX4s) -> Mux/4
  Wave particle velocity at the center of Appendages/5(uwXBs) -> Mux/5
  Mux/1 -> uwXis/1
  Wave particle velocity at hull CG/1(uwsCG) -> uwsCG/1
  Hydrostatic Forces and Moments/1(Out1) -> B_FM/1
  Constant6/1 -> Hydrostatic Forces and Moments/6(rho)
  Constant7/1 -> Hydrostatic Forces and Moments/7(g)
  Add/1 -> Hydrostatic Forces and Moments/8(Zb)
  Constant2/1 -> Add/1
  Constant1/1 -> Add/2
  dX_CTRL/1 -> Hydrostatic Forces and Moments/9(dX_CTRL)
  Wave Properties/1(L_wave) -> [L_wave]
  Wave Properties/2(A_wave) -> [A_wave]
  Wave Properties/3(k_wave) -> [k_wave]  "k"
  Wave Properties/4(w_wave) -> [w_wave]  "w"
  [A_wave] -> Hydrostatic Forces and Moments/3(A_wave)
  [k_wave] -> Hydrostatic Forces and Moments/4(k_wave)
  [w_wave] -> Hydrostatic Forces and Moments/5(w_wave)
  [L_wave] -> Sectional Wave Particle & Rigid Body Velocities/8(L_wave)
  [A_wave] -> Sectional Wave Particle & Rigid Body Velocities/9(A_wave)
  [k_wave] -> Sectional Wave Particle & Rigid Body Velocities/10(k_wave)
  [w_wave] -> Sectional Wave Particle & Rigid Body Velocities/11(w_wave)
  [k_wave] -> Local eff. Depth/3(k_wave)
  [A_wave] -> Local eff. Depth/5(a_wave)
  [w_wave] -> Local eff. Depth/4(w_wave)
  [L_wave] -> Wave particle velocity at hull CG/4(L_wave)
  [A_wave] -> Wave particle velocity at hull CG/7(A_wave)
  [k_wave] -> Wave particle velocity at hull CG/8(k_wave)
  [w_wave] -> Wave particle velocity at hull CG/9(w_wave)
  [L_wave] -> Wave particle velocity at the center of Appendages/9(L_wave)
  [A_wave] -> Wave particle velocity at the center of Appendages/12(A_wave)
  [k_wave] -> Wave particle velocity at the center of Appendages/13(k_wave)
  [w_wave] -> Wave particle velocity at the center of Appendages/14(w_wave)
  Clock/1 -> [time]
  [time] -> Sectional Wave Particle & Rigid Body Velocities/1(time)
  [time] -> Hydrostatic Forces and Moments/1(time)
  [time] -> Local eff. Depth/1(time)
  [time] -> Wave particle velocity at hull CG/1(time)
  [time] -> Wave particle velocity at the center of Appendages/1(time)
  U_ship/1 -> [U_ship]
  [U_ship] -> Sectional Wave Particle & Rigid Body Velocities/2(U_ship)
  [U_ship] -> Wave particle velocity at the center of Appendages/8(U_ship)
  phi_wave/1 -> [phi_wave]
  beta_wave/1 -> [beta_wave]
  [phi_wave] -> Sectional Wave Particle & Rigid Body Velocities/6(phi_wave)
  [beta_wave] -> Sectional Wave Particle & Rigid Body Velocities/7(beta_wave)
  [phi_wave] -> Wave particle velocity at hull CG/5(phi_wave)
  [beta_wave] -> Wave particle velocity at hull CG/6(beta_wave)
  [phi_wave] -> Wave particle velocity at the center of Appendages/10(phi_wave)
  [beta_wave] -> Wave particle velocity at the center of Appendages/11(beta_wave)

== system Model_6DOF/HDM/HDM B3/X/X'dXi ==
  UeX : Inport
  dXeff : Inport  Port=2
  Gain : Gain  Gain=-1
  Gain{4..7} (4 alike) : Gain
  Mux : Mux  Inputs=5
  Saturation6 : Saturate  UpperLimit=-1.543332  LowerLimit=-5.14444
  Selector10 : Selector  InputPortWidth=5  IndexOptions=Index vector (dialog)  Indices=4  OutputSizes=1
  Selector11 : Selector  InputPortWidth=5  IndexOptions=Index vector (dialog)  Indices=4  OutputSizes=1
  Selector12 : Selector  InputPortWidth=5  IndexOptions=Index vector (dialog)  Indices=5  OutputSizes=1
  Selector2 : Selector  InputPortWidth=5  IndexOptions=Index vector (dialog)  Indices=5  OutputSizes=1
  Selector4 : Selector  InputPortWidth=5  IndexOptions=Index vector (dialog)  Indices=1  OutputSizes=1
  Selector5 : Selector  InputPortWidth=5  IndexOptions=Index vector (dialog)  Indices=1  OutputSizes=1
  Selector6 : Selector  InputPortWidth=5  IndexOptions=Index vector (dialog)  Indices=2  OutputSizes=1
  Selector7 : Selector  InputPortWidth=5  IndexOptions=Index vector (dialog)  Indices=2  OutputSizes=1
  Selector8 : Selector  InputPortWidth=5  IndexOptions=Index vector (dialog)  Indices=3  OutputSizes=1
  Selector9 : Selector  InputPortWidth=5  IndexOptions=Index vector (dialog)  Indices=3  OutputSizes=1
  To Workspace : ToWorkspace  VariableName=UeX  SaveFormat=Timeseries  SampleTime=-1
  XudX1 : Lookup_n-D  BreakpointsForDimension1=[-30 -20 -10 0 10 20 30]  BreakpointsForDimension2=|  Table=|  InternalRulePriority=Speed  RndMeth=Simplest
      BreakpointsForDimension2=|
      | [-7.716666
      | -5.144444
      | -3.0866664
      | -1.5433332
      | ]
      Table=|
      | reshape([3.2151E-04
      | 1.4055E-04
      | 2.3723E-05
      | -2.9685E-05
      | 2.3777E-05
      | 1.3375E-04
      | 3.3722E-04
      | 1.6076E-04
      | 7.0275E-05
      | 1.1862E-05
      | -1.4843E-05
      | 1.1889E-05
      | 6.6875E-05
      | 1.6861E-04
      | 1.6698E-04
      | 6.8790E-05
      | 1.2322E-05
      | -1.4312E-05
      | 1.2274E-05
      | 6.7265E-05
      | 1.7083E-04
      | 3.4224E-04
      | 1.3333E-04
      | 2.5937E-05
      | -6.5668E-05
      | 2.5937E-05
      | 1.3102E-04
      | 3.4214E-04
      | ],[7,4])
      settings: InputPortMap=u0,u1
  XudX2 : Lookup_n-D  BreakpointsForDimension1=[-30 -20 -10 0 10 20 30]  BreakpointsForDimension2=|  Table=|  InternalRulePriority=Speed  RndMeth=Simplest
      BreakpointsForDimension2=|
      | [-7.716666
      | -5.144444
      | -3.0866664
      | -1.5433332
      | ]
      Table=|
      | reshape([2.9233E-04
      | 1.3189E-04
      | 2.3224E-05
      | -2.9022E-05
      | 1.9675E-05
      | 1.4726E-04
      | 3.7676E-04
      | 1.4617E-04
      | 6.5945E-05
      | 1.1612E-05
      | -1.4511E-05
      | 9.8375E-06
      | 7.3630E-05
      | 1.8838E-04
      | 1.7319E-04
      | 6.7285E-05
      | 1.2060E-05
      | -2.5958E-05
      | 1.0337E-05
      | 7.6660E-05
      | 1.8963E-04
      | 3.4748E-04
      | 1.3335E-04
      | 2.2395E-05
      | -2.6403E-05
      | 2.2395E-05
      | 1.5181E-04
      | 3.8598E-04
      | ],[7,4])
      settings: InputPortMap=u0,u1
  XudX3 : Lookup_n-D  BreakpointsForDimension1=[-30 -20 -10 0 10 20 30]  BreakpointsForDimension2=|  Table=|  InternalRulePriority=Speed  RndMeth=Simplest
      BreakpointsForDimension2=|
      | [-7.716666
      | -5.144444
      | -3.0866664
      | -1.5433332
      | ]
      Table=|
      | reshape([3.5642E-04
      | 1.5674E-04
      | 2.5449E-05
      | -2.9060E-05
      | 2.6726E-05
      | 1.6225E-04
      | 3.1115E-04
      | 1.7821E-04
      | 7.8370E-05
      | 1.2725E-05
      | -1.4530E-05
      | 1.3363E-05
      | 8.1125E-05
      | 1.5558E-04
      | 1.9053E-04
      | 8.0600E-05
      | 1.2911E-05
      | -1.3998E-05
      | 1.3672E-05
      | 7.4645E-05
      | 1.6290E-04
      | 3.8447E-04
      | 1.4526E-04
      | 2.7824E-05
      | -2.6434E-05
      | 2.7824E-05
      | 1.5039E-04
      | 3.2499E-04
      | ],[7,4])
      settings: InputPortMap=u0,u1
  XudX4 : Lookup_n-D  BreakpointsForDimension1=[-30 -20 -10 0 10 20 30]  BreakpointsForDimension2=|  Table=|  InternalRulePriority=Speed  RndMeth=Simplest
      BreakpointsForDimension2=|
      | [-7.716666
      | -5.144444
      | -3.0866664
      | -1.5433332
      | ]
      Table=|
      | reshape([3.4525E-04
      | 1.3840E-04
      | 2.4668E-05
      | -2.9702E-05
      | 2.4205E-05
      | 1.2737E-04
      | 3.2790E-04
      | 1.7263E-04
      | 6.9200E-05
      | 1.2334E-05
      | -1.4851E-05
      | 1.2103E-05
      | 6.3685E-05
      | 1.6395E-04
      | 1.7298E-04
      | 6.9435E-05
      | 1.2696E-05
      | -1.4315E-05
      | 1.2608E-05
      | 6.9175E-05
      | 1.6779E-04
      | 3.3803E-04
      | 1.5513E-04
      | 2.6677E-05
      | -2.7052E-05
      | 2.6677E-05
      | 1.3644E-04
      | 3.3780E-04
      | ],[7,4])
      settings: InputPortMap=u0,u1
  XudXB : Lookup_n-D  BreakpointsForDimension1=[-30 -20 -10 0 10 20 30]  BreakpointsForDimension2=[-5.14444 -3.08666664 -1.54332]  Table=|  InternalRulePriority=Speed  RndMeth=Simplest
      | reshape([6.9060E-04
      | 3.9256E-04
      | 1.5651E-04
      | 0.0000E+00
      | 1.1449E-04
      | 4.2412E-04
      | 5.7370E-04
      | 6.4542E-04
      | 3.9138E-04
      | 1.5593E-04
      | 0.0000E+00
      | 1.1381E-04
      | 4.1205E-04
      | 5.6813E-04
      | 6.5675E-04
      | 3.9410E-04
      | 1.1271E-04
      | 0.0000E+00
      | 1.1271E-04
      | 4.2649E-04
      | 5.7604E-04
      | ],[7,3])
      settings: InputPortMap=u0,u1
  Out1 : Outport
  wires:
  Selector2/1 -> XudXB/1
  XudX4/1 -> Gain7/1
  XudX3/1 -> Gain5/1
  XudX2/1 -> Gain6/1
  XudX1/1 -> Gain4/1
  Mux/1 -> Out1/1
  dXeff/1 -> Selector2/1, Selector10/1, Selector8/1, Selector6/1, Selector4/1
  Selector4/1 -> XudX1/1
  Selector5/1 -> XudX1/2
  Selector6/1 -> XudX2/1
  Selector7/1 -> XudX2/2
  Selector8/1 -> XudX3/1
  Selector9/1 -> XudX3/2
  UeX/1 -> Gain/1
  Selector11/1 -> XudX4/2
  Selector10/1 -> XudX4/1
  Selector12/1 -> XudXB/2
  Gain4/1 -> Mux/1
  Gain6/1 -> Mux/2
  Gain5/1 -> Mux/3
  Gain7/1 -> Mux/4
  XudXB/1 -> Mux/5
  Gain/1 -> To Workspace/1, Saturation6/1
  Saturation6/1 -> Selector11/1, Selector12/1, Selector9/1, Selector7/1, Selector5/1

== system Model_6DOF/HDM/HDM B3/Y/YdXi ==
  dX : Inport
  z : Inport  Port=2
  Mux : Mux
  Selector1 : Selector  InputPortWidth=5  IndexOptions=Index vector (dialog)  Indices=2  OutputSizes=1
  Selector2 : Selector  InputPortWidth=5  IndexOptions=Index vector (dialog)  Indices=3  OutputSizes=1
  Selector3 : Selector  InputPortWidth=5  IndexOptions=Index vector (dialog)  Indices=4  OutputSizes=1
  Selector7 : Selector  InputPortWidth=5  IndexOptions=Index vector (dialog)  Indices=1  OutputSizes=1
  YdX1 : Lookup_n-D  BreakpointsForDimension1=[-10 0 10]  BreakpointsForDimension2=|  BreakpointsForDimension3=[-5.14444 -3.08666664 -1.54332]  Table=|  InternalRulePriority=Speed  RndMeth=Simplest
      BreakpointsForDimension2=|
      | [-36.4062987
      | -18.4062987
      | -15.4062987
      | -13.9062987]
      Table=|
      | reshape([-1.8282E-04
      | -6.0037E-06
      | 1.6496E-04
      | -1.7978E-04
      | -2.4314E-06
      | 1.6969E-04
      | -1.4480E-04
      | -2.4314E-06
      | 2.0267E-04
      | -1.7641E-04
      | 1.4850E-06
      | 1.7514E-04],[3,4])
      settings: InputPortMap=u0,u1
  YdX2 : Lookup_n-D  BreakpointsForDimension1=[-10 0 10]  BreakpointsForDimension2=|  BreakpointsForDimension3=[-5.14444 -3.08666664 -1.54332]  Table=|  InternalRulePriority=Speed  RndMeth=Simplest
      BreakpointsForDimension2=|
      | [-36.4062987
      | -18.4062987
      | -15.4062987
      | -13.9062987]
      Table=|
      | reshape([1.4857E-04
      | -6.6611E-06
      | -1.5932E-04
      | 1.4200E-04
      | -1.2968E-05
      | -1.6860E-04
      | 9.4982E-05
      | -1.2968E-05
      | -2.1344E-04
      | 1.3366E-04
      | -2.3176E-05
      | -1.8599E-04],[3,4])
      settings: InputPortMap=u0,u1
  YdX3 : Lookup_n-D  BreakpointsForDimension1=[-10 0 10]  BreakpointsForDimension2=|  BreakpointsForDimension3=[-5.14444 -3.08666664 -1.54332]  Table=|  InternalRulePriority=Speed  RndMeth=Simplest
      BreakpointsForDimension2=|
      | [-36.4062987
      | -18.4062987
      | -15.4062987
      | -13.9062987]
      Table=|
      | reshape([2.0207E-04
      | 6.9701E-06
      | -1.9141E-04
      | 2.0588E-04
      | 1.3213E-05
      | -1.8007E-04
      | 2.2753E-04
      | 1.3213E-05
      | -1.0937E-04
      | 2.1222E-04
      | 2.3270E-05
      | -1.6161E-04],[3,4])
      settings: InputPortMap=u0,u1
  YdX4 : Lookup_n-D  BreakpointsForDimension1=[-10 0 10]  BreakpointsForDimension2=|  BreakpointsForDimension3=[-5.14444 -3.08666664 -1.54332]  Table=|  InternalRulePriority=Speed  RndMeth=Simplest
      BreakpointsForDimension2=|
      | [-36.4062987
      | -18.4062987
      | -15.4062987
      | -13.9062987]
      Table=|
      | reshape([-1.7022E-04
      | 5.9932E-06
      | 1.8722E-04
      | -1.7390E-04
      | 2.3770E-06
      | 1.8293E-04
      | -2.0489E-04
      | 2.3770E-06
      | 1.4658E-04
      | -1.7771E-04
      | -1.6689E-06
      | 1.7805E-04],[3,4])
      settings: InputPortMap=u0,u1
  YdX : Outport
  wires:
  Mux/1 -> YdX/1
  z/1 -> YdX4/2, YdX3/2, YdX2/2, YdX1/2
  YdX1/1 -> Mux/1
  YdX2/1 -> Mux/2
  YdX3/1 -> Mux/3
  YdX4/1 -> Mux/4
  Selector7/1 -> YdX1/1
  dX/1 -> Selector2/1, Selector3/1, Selector1/1, Selector7/1
  Selector3/1 -> YdX4/1
  Selector2/1 -> YdX3/1
  Selector1/1 -> YdX2/1

== system Model_6DOF/HDM/HDM B3/Z/ZdXi ==
  dX : Inport
  z : Inport  Port=2
  Demux6 : Demux  Outputs=5
  Mux : Mux  Inputs=5
  ZudX1 q+10 : Lookup_n-D  BreakpointsForDimension1=[-30 -20 -10 0 10 20 30]  BreakpointsForDimension2=[-35.0624 -15.3724 -13.8724]  BreakpointsForDimension3=[-35.0624 -15.3724 -13.8724]  Table=|  InternalRulePriority=Speed  RndMeth=Simplest
      | reshape([-0.003226964
      | -0.002116041
      | -0.001005119
      | 0.000105803
      | 0.001216725
      | 0.002327647
      | 0.003438569
      | -0.003036597
      | -0.001876165
      | -0.000715732
      | 0.0004447
      | 0.001605132
      | 0.002765565
      | 0.003925997
      | -0.003676642
      | -0.002490275
      | -0.001303908
      | -0.000117541
      | 0.001068826
      | 0.002255193
      | 0.00344156],[7,3])
      settings: InputPortMap=u0,u1
  ZudX1 q+6 : Lookup_n-D  BreakpointsForDimension1=[-30 -20 -10 0 10 20 30]  BreakpointsForDimension2=[-35.0624 -15.3724 -13.8724]  BreakpointsForDimension3=[-5.14444 -3.08666664 -1.54332]  Table=|  InternalRulePriority=Speed  RndMeth=Simplest
      | reshape([-0.001383757
      | -0.000911
      | -0.000438243
      | 3.45135E-05
      | 0.00050727
      | 0.000980027
      | 0.001452784
      | -0.001383757
      | -0.000911
      | -0.000438243
      | 3.45135E-05
      | 0.00050727
      | 0.000980027
      | 0.001452784
      | -0.001353354
      | -0.000887631
      | -0.000421908
      | 4.38143E-05
      | 0.000509537
      | 0.00097526
      | 0.001440982],[7,3])
      settings: InputPortMap=u0,u1
  ZudX1 q+7 : Lookup_n-D  BreakpointsForDimension1=[-30 -20 -10 0 10 20 30]  BreakpointsForDimension2=[-35.0624 -15.3724 -13.8724]  BreakpointsForDimension3=[-5.14444 -3.08666664 -1.54332]  Table=|  InternalRulePriority=Speed  RndMeth=Simplest
      | reshape([-0.001358511
      | -0.00091651
      | -0.000474508
      | -3.25062E-05
      | 0.000409495
      | 0.000851497
      | 0.001293499
      | -0.001303275
      | -0.00086798
      | -0.000432686
      | 2.60877E-06
      | 0.000437903
      | 0.000873198
      | 0.001308493
      | -0.001263287
      | -0.000836064
      | -0.00040884
      | 1.83841E-05
      | 0.000445608
      | 0.000872832
      | 0.001300056],[7,3])
      settings: InputPortMap=u0,u1
  ZudX1 q+8 : Lookup_n-D  BreakpointsForDimension1=[-30 -20 -10 0 10 20 30]  BreakpointsForDimension2=[-35.0624 -15.3724 -13.8724]  BreakpointsForDimension3=[-5.14444 -3.08666664 -1.54332]  Table=|  InternalRulePriority=Speed  RndMeth=Simplest
      | reshape([0.001309084
      | 0.000864124
      | 0.000419163
      | -2.5798E-05
      | -0.000470759
      | -0.000915719
      | -0.00136068
      | 0.001321953
      | 0.000882434
      | 0.000442915
      | 3.39516E-06
      | -0.000436124
      | -0.000875644
      | -0.001315163
      | 0.001313186
      | 0.000881448
      | 0.000449709
      | 1.79712E-05
      | -0.000413767
      | -0.000845505
      | -0.001277243],[7,3])
      settings: InputPortMap=u0,u1
  ZudX1 q+9 : Lookup_n-D  BreakpointsForDimension1=[-30 -20 -10 0 10 20 30]  BreakpointsForDimension2=[-35.0624 -15.3724 -13.8724]  BreakpointsForDimension3=[-5.14444 -3.08666664 -1.54332]  Table=|  InternalRulePriority=Speed  RndMeth=Simplest
      | reshape([0.001464336
      | 0.000977857
      | 0.000491377
      | 4.89775E-06
      | -0.000481582
      | -0.000968061
      | -0.00145454
      | 0.001455937
      | 0.00098192
      | 0.000507903
      | 3.38863E-05
      | -0.00044013
      | -0.000914147
      | -0.001388164
      | 0.001460604
      | 0.00098818
      | 0.000515756
      | 4.33325E-05
      | -0.000429091
      | -0.000901515
      | -0.001373939],[7,3])
      settings: InputPortMap=u0,u1
  ZdX : Outport
  wires:
  ZudX1 q+9/1 -> Mux/4
  ZudX1 q+8/1 -> Mux/3
  ZudX1 q+7/1 -> Mux/2
  ZudX1 q+6/1 -> Mux/1
  ZudX1 q+10/1 -> Mux/5
  z/1 -> ZudX1 q+9/2, ZudX1 q+10/2, ZudX1 q+8/2, ZudX1 q+7/2, ZudX1 q+6/2
  Demux6/5 -> ZudX1 q+10/1
  Mux/1 -> ZdX/1
  Demux6/1 -> ZudX1 q+6/1
  Demux6/2 -> ZudX1 q+7/1
  Demux6/4 -> ZudX1 q+9/1
  dX/1 -> Demux6/1
  Demux6/3 -> ZudX1 q+8/1
